simulink model "Control_v6_PID"  (R2020b)
settings: Solver=FixedStepAuto  StartTime=0.0  StopTime=t_sim  FixedStep=TimeStep  RelTol=1e-3
values from neighbouring files (symbols this model uses):
  date_IGRF = [date.year,date.month,date.day]    [main_SCA_v3.m]    (also in main_SCA_v3_alt.m; main_SCA_v4_LQR.m; main_SCA_v5.m)
  nmax = 2    [main_SCA.m]    (also in main_SCA_v3.m; main_SCA_v3_alt.m; main_SCA_v4_LQR.m; main_SCA_v5.m)
  Use_IGRF = 0    [main_SCA.m]    (also in main_SCA_v3.m; main_SCA_v3_alt.m; main_SCA_v4_LQR.m; main_SCA_v5.m = 1)
undefined symbols (not defined in the file or in its folder): att, date, deg, DipoleMod, DiscIntNeverNeededParam, IonSataero, km, orbit, rad, s, sat
libraries: vrlib x20, aerolibconvert2 x14, aerolibutil x14, dspmathops x13, sharedtransform x12, simulink x5, simulink_extras x2, dspstat3 x1, aerolibatmos2 x1, aerolibobsolete x1, sharedutil x1, aerolibcelestial x1
(part 1 of 3)
settings Model: EnablePacing=on  PacingRate=1000  Creator=colpari  LastModifiedBy=kang Shinok
settings OptimizationCC: DefaultParameterBehavior=Inlined  UseDivisionForNetSlopeComputation=on  GainParamInheritBuiltInType=on  UseFloatMulNetSlope=on  InlineInvariantSignals=on  EfficientFloat2IntCast=on  LifeSpan=1
settings HardwareCC: ProdLongLongMode=on
settings SFSimCC: MATLABDynamicMemAlloc=off
settings RTWCC: GenerateReport=on  LaunchReport=on
settings CodeAppCC: ForceParamTrailComments=on
settings GRTTargetCC: CombineSignalStateStructs=on  MatFileLogging=off  SupportVariableSizeSignals=on

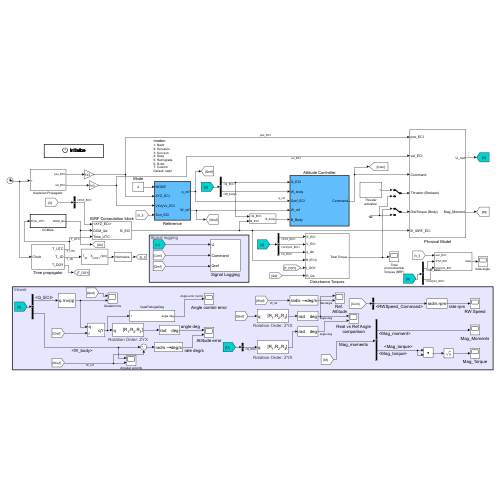
[thumbnail: Simulink's stored preview of the top-level diagram]
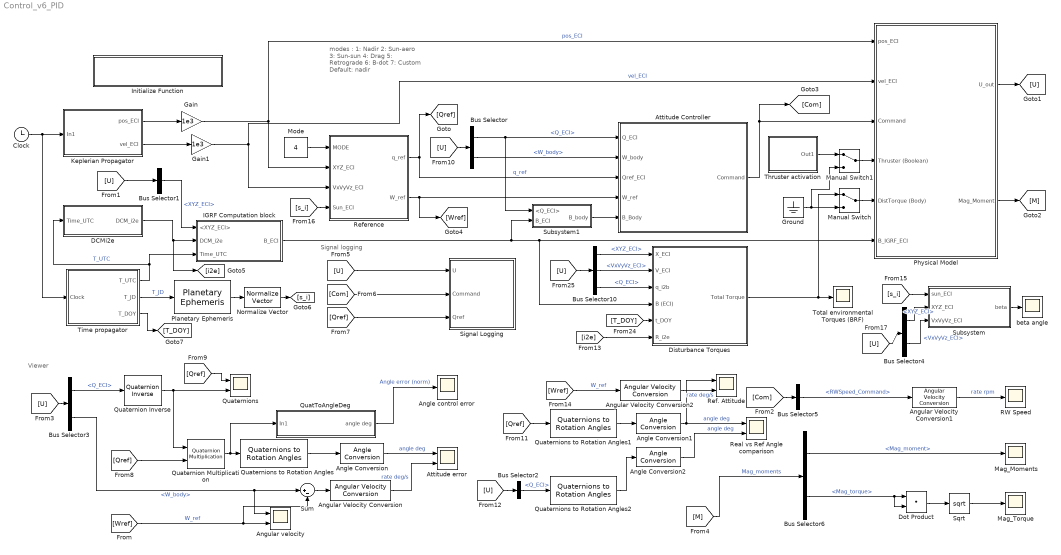
== system Control_v6_PID ==
  note: Viewer
  note: Signal logging
  note: modes :
      | 1: Nadir
      | 2: Sun-aero
      | 3: Sun-sun
      | 4: Drag
      | 5: Retrograde
      | 6: B-dot
      | 7: Custom
      | Default: nadir
  Angle Conversion : aerolibconvert2/Angle Conversion  IU=rad  OU=deg
  Angle Conversion1 : aerolibconvert2/Angle Conversion  IU=rad  OU=deg
  Angle Conversion2 : aerolibconvert2/Angle Conversion  IU=rad  OU=deg
  Angle control error : Scope
  Angular Velocity Conversion : aerolibconvert2/Angular Velocity Conversion  IU=rad/s  OU=deg/s
  Angular Velocity Conversion1 : aerolibconvert2/Angular Velocity Conversion  IU=rad/s  OU=rpm
  Angular Velocity Conversion2 : aerolibconvert2/Angular Velocity Conversion  IU=rad/s  OU=deg/s
  Angular velocity : Scope  NumInputPorts=2
  Attitude Controller : Subsystem  TreatAsAtomicUnit=on
  Attitude error : Scope  NumInputPorts=2
  Bus Selector : BusSelector  OutputSignals=Q_ECI,W_body
  Bus Selector1 : BusSelector  OutputSignals=XYZ_ECI
  Bus Selector10 : BusSelector  OutputSignals=XYZ_ECI,VxVyVz_ECI,Q_ECI
  Bus Selector2 : BusSelector  OutputSignals=Q_ECI
  Bus Selector3 : BusSelector  OutputSignals=Q_ECI,W_body
  Bus Selector4 : BusSelector  OutputSignals=XYZ_ECI,VxVyVz_ECI
  Bus Selector5 : BusSelector  OutputSignals=RWSpeed_Command
  Bus Selector6 : BusSelector  OutputSignals=Mag_moment,Mag_torque
  Clock : Clock
  DCMi2e : Subsystem  TreatAsAtomicUnit=on  SystemSampleTime=1
  Disturbance Torques : Subsystem
  Dot Product : DotProduct  InputSameDT=on  OutDataTypeStr=Inherit: Inherit via internal rule
  Gain : Gain  Gain=1e3
  Gain1 : Gain  Gain=1e3
  Ground : Ground
  IGRF Computation block : Subsystem
  Initialize Function : Subsystem  TreatAsAtomicUnit=on
  Keplerian Propagator : Subsystem
  Mag_Moments : Scope
  Mag_Torque : Scope
  Manual Switch : ManualSwitch
  Manual Switch1 : ManualSwitch
  Mode : Constant  Value=4  OutDataTypeStr=int8
  Normalize Vector : vrlib/Utilities/Normalize Vector  maxzero=0
  Physical Model : Subsystem
      settings: MinAlgLoopOccurrences=on
  Planetary Ephemeris : aerolibcelestial/Planetary Ephemeris  kmflag=km,km/s  epochflag=Julian date  de=DE405  nCenter=Earth  nTarget=Sun  errorflag=Error  velflag=off
      settings: SourceProductBaseCode=AE
  QuatToAngleDeg : Subsystem
  Quaternion Inverse : aerolibutil/Quaternion Inverse
  Quaternion Multiplication : aerolibutil/Quaternion Multiplication
  Quaternions : Scope  NumInputPorts=2
  Quaternions to Rotation Angles : sharedtransform/Quaternions to Rotation Angles  rotationOrder=ZYX  aMode=aMode
      settings: SourceProductBaseCode=AE,PW,DR,MT,UV,VE
  Quaternions to Rotation Angles1 : sharedtransform/Quaternions to Rotation Angles  rotationOrder=ZYX  aMode=aMode
      settings: SourceProductBaseCode=AE,PW,DR,MT,UV,VE
  Quaternions to Rotation Angles2 : sharedtransform/Quaternions to Rotation Angles  rotationOrder=ZYX  aMode=aMode
      settings: SourceProductBaseCode=AE,PW,DR,MT,UV,VE
  RW Speed : Scope
  Real vs Ref Angle comparison : Scope  NumInputPorts=2
  Ref. Attitude : Scope  NumInputPorts=2
  Reference : Subsystem  TreatAsAtomicUnit=on
  Signal Logging : Subsystem
  Sqrt : Sqrt  SaturateOnIntegerOverflow=on
  Subsystem : Subsystem
  Subsystem1 : Subsystem
  Sum : Sum  Inputs=|+-
  Thruster activation : Subsystem
  Time propagator : Subsystem
  Total environmental Torques (BRF) : Scope
  beta angle : Scope
  wires:
  Clock/1 -> Keplerian Propagator/1(In1), Time propagator/1(Clock)
  Keplerian Propagator/1(pos_ECI) -> Gain/1
  Keplerian Propagator/2(vel_ECI) -> Gain1/1
  Planetary Ephemeris/1 -> Normalize Vector/1
  Time propagator/2(T_JD) -> Planetary Ephemeris/1  "T_JD"
  Reference/1(q_ref) -> [Qref], Attitude Controller/3(Qref_ECI)  "q_ref"
  Physical Model/1(U_out) -> [U]
  Time propagator/1(T_UTC) -> DCMi2e/1(Time_UTC), IGRF Computation block/3("Time_UTC ")  "T_UTC"
  Gain/1 -> Reference/2(XYZ_ECI), Physical Model/1(pos_ECI)  "pos_ECI"
  Gain1/1 -> Reference/3(VxVyVz_ECI), Physical Model/2(vel_ECI)  "vel_ECI"
  Attitude Controller/1(Command) -> Physical Model/3(Command), [Com]
  IGRF Computation block/1(B_ECI) -> Subsystem1/2(B_ECI), Disturbance Torques/4(B (ECI)), Physical Model/6(B_IGRF_ECI)
  [U] -> Bus Selector/1
  Bus Selector/1 -> Subsystem1/1(<Q_ECI>), Attitude Controller/1(Q_ECI)  "<Q_ECI>"
  Bus Selector/2 -> Attitude Controller/2(W_body)  "<W_body>"
  [U] -> Bus Selector1/1
  Bus Selector1/1 -> IGRF Computation block/1(<XYZ_ECI>)  "<XYZ_ECI>"
  [Qref] -> Signal Logging/3(Qref)
  Quaternions to Rotation Angles/1 -> Angle Conversion/1
  Bus Selector6/2 -> Dot Product/2, Dot Product/1  "<Mag_torque>"
  Bus Selector6/1 -> Mag_Moments/1  "<Mag_moment>"
  Dot Product/1 -> Sqrt/1
  Bus Selector3/1 -> Quaternion Inverse/1  "<Q_ECI>"
  Sqrt/1 -> Mag_Torque/1
  Bus Selector5/1 -> Angular Velocity Conversion1/1  "<RWSpeed_Command>"
  [Com] -> Signal Logging/2(Command)
  [Com] -> Bus Selector5/1
  Bus Selector3/2 -> Sum/1, Angular velocity/1  "<W_body>"
  [Qref] -> Quaternion Multiplication/2
  [U] -> Bus Selector3/1
  Quaternion Inverse/1 -> Quaternion Multiplication/1, Quaternions/2
  [M] -> Bus Selector6/1  "Mag_moments"
  Angular Velocity Conversion/1 -> Attitude error/2  "rate deg/s"
  Quaternion Multiplication/1 -> QuatToAngleDeg/1(In1), Quaternions to Rotation Angles/1
  [U] -> Signal Logging/1(U)
  Angle Conversion/1 -> Attitude error/1  "angle deg"
  Angular Velocity Conversion1/1 -> RW Speed/1  "rate rpm"
  Physical Model/2(Mag_Moment) -> [M]
  Subsystem1/1(B_body) -> Attitude Controller/5(B_Body)
  QuatToAngleDeg/1(angle deg) -> Angle control error/1  "Angle error (norm)"
  [Qref] -> Quaternions/1
  Reference/2(W_ref) -> [Wref], Attitude Controller/4(W_ref)
  [Wref] -> Sum/2, Angular velocity/2  "W_ref"
  Sum/1 -> Angular Velocity Conversion/1
  [Qref] -> Quaternions to Rotation Angles1/1
  Angle Conversion1/1 -> Ref. Attitude/1, Real vs Ref Angle comparison/1  "angle deg"
  Quaternions to Rotation Angles1/1 -> Angle Conversion1/1
  Thruster activation/1(Out1) -> Manual Switch1/1
  [U] -> Bus Selector10/1
  [T_DOY] -> Disturbance Torques/5(t_DOY)
  Bus Selector10/3 -> Disturbance Torques/3(q_i2b)  "<Q_ECI>"
  Time propagator/3(T_DOY) -> [T_DOY]
  Disturbance Torques/1("Total Torque ") -> Total environmental Torques (BRF)/1, Manual Switch/1
  Manual Switch/1 -> Physical Model/5(DistTorque (Body))
  Ground/1 -> Manual Switch/2, Manual Switch1/2
  Bus Selector2/1 -> Quaternions to Rotation Angles2/1  "<Q_ECI>"
  Quaternions to Rotation Angles2/1 -> Angle Conversion2/1
  Angle Conversion2/1 -> Real vs Ref Angle comparison/2  "angle deg"
  [U] -> Bus Selector2/1
  [Wref] -> Angular Velocity Conversion2/1  "W_ref"
  Angular Velocity Conversion2/1 -> Ref. Attitude/2  "rate deg/s"
  DCMi2e/1(DCM_i2e) -> [i2e], IGRF Computation block/2("DCM_i2e ")
  [i2e] -> Disturbance Torques/6(R_i2e)
  Bus Selector10/1 -> Disturbance Torques/1(X_ECI)  "<XYZ_ECI>"
  Bus Selector10/2 -> Disturbance Torques/2(V_ECI)  "<VxVyVz_ECI>"
  Manual Switch1/1 -> Physical Model/4(Thruster (Boolean))
  Mode/1 -> Reference/1(MODE)
  [s_i] -> Subsystem/1(sun_ECI)
  Subsystem/1(beta) -> beta angle/1
  Normalize Vector/1 -> [s_i]
  [s_i] -> Reference/4(Sun_ECI)
  [U] -> Bus Selector4/1
  Bus Selector4/1 -> Subsystem/2(XYZ_ECI)  "<XYZ_ECI>"
  Bus Selector4/2 -> Subsystem/3(VxVyVz_ECI)  "<VxVyVz_ECI>"

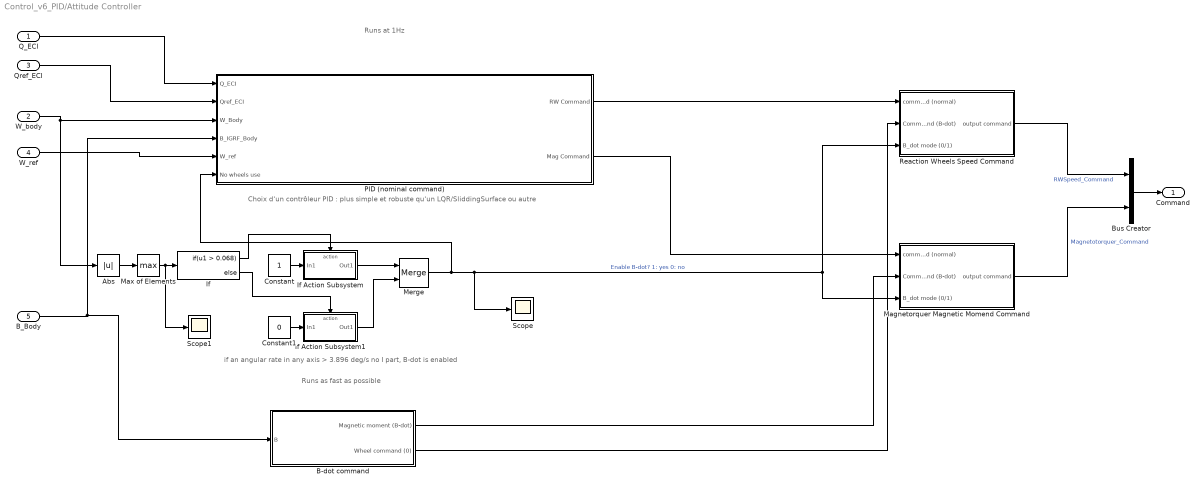
== system Control_v6_PID/Attitude Controller ==
  note: Choix d'un contrôleur PID : plus simple et robuste qu'un LQR/SliddingSurface ou autre
  note: Runs as fast as possible
  note: Runs at 1Hz
  note: if an angular rate in any axis > 3.896 deg/s no I part, B-dot is enabled
  Q_ECI : Inport
  W_body : Inport  Port=2
  Qref_ECI : Inport  Port=3
  W_ref : Inport  Port=4
  B_Body : Inport  Port=5
  Abs : Abs
  B-dot command : Subsystem  TreatAsAtomicUnit=on
  Bus Creator : BusCreator  Inputs=2
  Constant : Constant
  Constant1 : Constant  Value=0
  If : If  IfExpression=u1 > 0.068
  If Action Subsystem : Subsystem  TreatAsAtomicUnit=on
  If Action Subsystem1 : Subsystem  TreatAsAtomicUnit=on
  Magnetorquer Magnetic Momend Command : Subsystem
  Max of Elements : MinMax  Function=max
  Merge : Merge
  PID (nominal command) : Subsystem  TreatAsAtomicUnit=on  SystemSampleTime=1
  Reaction Wheels Speed Command : Subsystem
  Scope : Scope
  Scope1 : Scope
  Command : Outport  VectorParamsAs1DForOutWhenUnconnected=off
  wires:
  B_Body/1 -> B-dot command/1(B), PID (nominal command)/4(B_IGRF_Body)
  Magnetorquer Magnetic Momend Command/1(output command) -> Bus Creator/2  "Magnetotorquer_Command"
  Reaction Wheels Speed Command/1(output command) -> Bus Creator/1  "RWSpeed_Command"
  B-dot command/2(Wheel command (0)) -> Reaction Wheels Speed Command/2(Command (B-dot))
  B-dot command/1(Magnetic moment (B-dot)) -> Magnetorquer Magnetic Momend Command/2(Command (B-dot))
  Q_ECI/1 -> PID (nominal command)/1(Q_ECI)
  Qref_ECI/1 -> PID (nominal command)/2(Qref_ECI)
  PID (nominal command)/1(RW Command) -> Reaction Wheels Speed Command/1(" command (normal)")
  PID (nominal command)/2(Mag Command) -> Magnetorquer Magnetic Momend Command/1(" command (normal)")
  Bus Creator/1 -> Command/1
  Abs/1 -> Max of Elements/1
  If/1 -> If Action Subsystem/Action
  If Action Subsystem1/1(Out1) -> Merge/2
  Max of Elements/1 -> Scope1/1, If/1
  If/2 -> If Action Subsystem1/Action
  If Action Subsystem/1(Out1) -> Merge/1
  Constant/1 -> If Action Subsystem/1(In1)
  Merge/1 -> Scope/1, Magnetorquer Magnetic Momend Command/3(B_dot mode (0/1)), Reaction Wheels Speed Command/3(B_dot mode (0/1)), PID (nominal command)/6(No wheels use)  "Enable B-dot? 1: yes 0: no"
  Constant1/1 -> If Action Subsystem1/1(In1)
  W_body/1 -> Abs/1, PID (nominal command)/3(W_Body)
  W_ref/1 -> PID (nominal command)/5(W_ref)

== system Control_v6_PID/DCMi2e ==
  note: Slower subsytem because it's too slow
  Time_UTC : Inport
  ECI to ECEF : MATLABFcn  MATLABFcn=eci2ecef  OutputDimensions=[3;3]  Output1D=off
  DCM_i2e : Outport
  wires:
  ECI to ECEF/1 -> DCM_i2e/1
  Time_UTC/1 -> ECI to ECEF/1

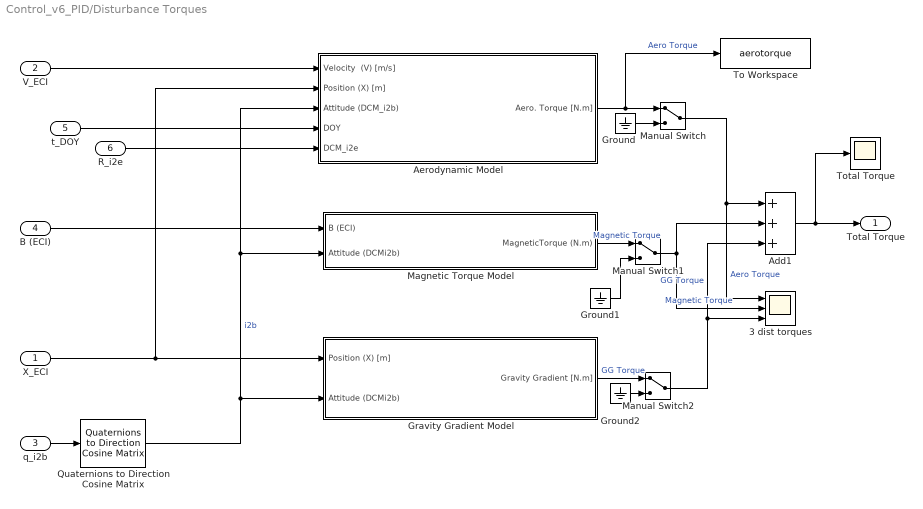
== system Control_v6_PID/Disturbance Torques ==
  X_ECI : Inport
  V_ECI : Inport  Port=2
  q_i2b : Inport  Port=3
  B (ECI) : Inport  Port=4
  t_DOY : Inport  Port=5
  R_i2e : Inport  Port=6
  3 dist torques : Scope  NumInputPorts=3
  Add1 : Sum  Inputs=+++
  Aerodynamic Model : Subsystem
  Gravity Gradient Model : Subsystem
  Ground : Ground
  Ground1 : Ground
  Ground2 : Ground
  Magnetic Torque Model : Subsystem
  Manual Switch : ManualSwitch
  Manual Switch1 : ManualSwitch
  Manual Switch2 : ManualSwitch
  Quaternions to Direction Cosine Matrix : sharedtransform/Quaternions to  Direction Cosine Matrix  aMode=aMode
      settings: SourceProductBaseCode=AE,PW,DR,MT,UV,VE
  To Workspace : ToWorkspace  VariableName=aerotorque  SaveFormat=Timeseries  SampleTime=-1
  Total Torque : Scope
  "Total Torque " : Outport
  wires:
  Add1/1 -> Total Torque/1, "Total Torque "/1
  V_ECI/1 -> Aerodynamic Model/1(Velocity  (V) [m/s])
  X_ECI/1 -> Aerodynamic Model/2(Position (X) [m]), Gravity Gradient Model/1("Position (X) [m] ")
  Manual Switch/1 -> 3 dist torques/1, Add1/1  "Aero Torque"
  Manual Switch2/1 -> Add1/3, 3 dist torques/3  "GG Torque"
  B (ECI)/1 -> Magnetic Torque Model/1(B (ECI))
  Manual Switch1/1 -> Add1/2, 3 dist torques/2  "Magnetic Torque"
  q_i2b/1 -> Quaternions to Direction Cosine Matrix/1
  Quaternions to Direction Cosine Matrix/1 -> Gravity Gradient Model/2(Attitude (DCMi2b)), Magnetic Torque Model/2(Attitude (DCMi2b)), Aerodynamic Model/3(Attitude (DCM_i2b))  "i2b"
  R_i2e/1 -> Aerodynamic Model/5(DCM_i2e)
  t_DOY/1 -> Aerodynamic Model/4(DOY)
  Ground/1 -> Manual Switch/2
  Aerodynamic Model/1(Aero. Torque [N.m]) -> To Workspace/1, Manual Switch/1  "Aero Torque"
  Magnetic Torque Model/1(MagneticTorque (N.m)) -> Manual Switch1/1  "Magnetic Torque"
  Ground1/1 -> Manual Switch1/2
  Ground2/1 -> Manual Switch2/2
  Gravity Gradient Model/1(Gravity Gradient [N.m]) -> Manual Switch2/1  "GG Torque"

== system Control_v6_PID/IGRF Computation block ==
  <XYZ_ECI> : Inport
  "DCM_i2e " : Inport  Port=2
  "Time_UTC " : Inport  Port=3
  Bus Creator : BusCreator  Inputs=5
  Bus Selector4 : BusSelector  OutputSignals=XYZ_ECI
  Constant : Constant  Value=[0.4;0.4;0.4]
  Cross Product : vrlib/Utilities/Cross Product
  Demux : Demux  Outputs=2
  ECI To LLA : MATLAB Function  TreatAsAtomicUnit=on
  MATLAB Function : MATLAB Function  TreatAsAtomicUnit=on
  Mux : Mux  Inputs=3
  Obtain B_ECI : Subsystem
  Product : Product  Multiplication=Matrix(*)
  Reshape : Reshape  OutputDimensionality=Row vector (2-D)
  Scope : Scope
  Terminator : Terminator
  To Workspace : ToWorkspace  VariableName=B_ECI  SaveFormat=Timeseries  SampleTime=-1
  B_ECI : Outport  VectorParamsAs1DForOutWhenUnconnected=off
  wires:
  ECI To LLA/3(long) -> Bus Creator/3
  ECI To LLA/2(lat) -> Bus Creator/2
  ECI To LLA/1(h) -> Bus Creator/1
  Demux/1 -> Bus Creator/4  "time_UTC"
  Demux/2 -> Terminator/1
  "DCM_i2e "/1 -> Product/2, Bus Creator/5  "DCM_i2e"
  <XYZ_ECI>/1 -> Bus Selector4/1
  Reshape/1 -> Product/1
  Product/1 -> ECI To LLA/1(X_ECEF)
  Bus Selector4/1 -> Reshape/1  "<XYZ_ECI>"
  Bus Creator/1 -> Obtain B_ECI/1(In1)
  Obtain B_ECI/1(u) -> Cross Product/2, MATLAB Function/1(u), Mux/1, To Workspace/1, B_ECI/1
  "Time_UTC "/1 -> Demux/1
  Mux/1 -> Scope/1
  MATLAB Function/1(y) -> Mux/2
  Constant/1 -> Cross Product/1
  Cross Product/1 -> Mux/3

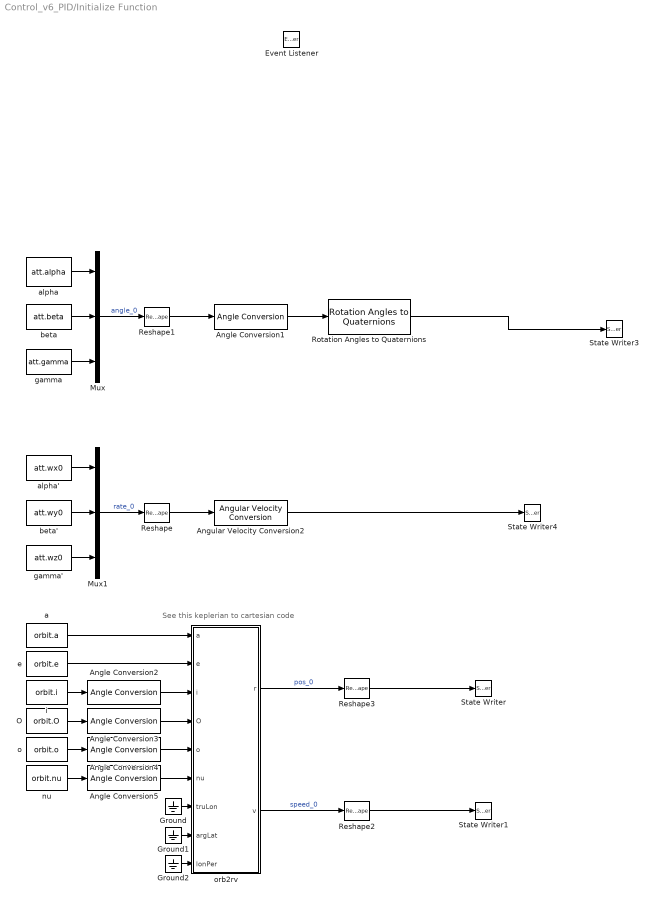
== system Control_v6_PID/Initialize Function ==
  note: See this keplerian to cartesian code
  Angle Conversion{1..5} (5 alike) : aerolibconvert2/Angle Conversion  IU=deg  OU=rad
  Angular Velocity Conversion2 : aerolibconvert2/Angular Velocity Conversion  IU=deg/s  OU=rad/s
  Event Listener : EventListener  DisableCoverage=on  EventName=reset
  Ground : Ground
  Ground1 : Ground
  Ground2 : Ground
  Mux : Mux  Inputs=3
  Mux1 : Mux  Inputs=3
  O : Constant  Value=orbit.O
  Reshape{,1..3} (4 alike) : Reshape  OutputDimensionality=Column vector (2-D)
  Rotation Angles to Quaternions : sharedtransform/Rotation Angles to Quaternions  rotationOrder=ZYX  aMode=aMode
      settings: SourceProductBaseCode=AE,PW,DR,MT,UV,VE
  State Writer : StateWriter  StateOwnerBlock=../../Keplerian Propagator/Integrator
  State Writer1 : StateWriter  StateOwnerBlock=../../Keplerian Propagator/Integrator1
  State Writer3 : StateWriter  StateOwnerBlock=../../Physical Model/6DOF in ECI frame/Compute Q_ECI/Integrator_quat
  State Writer4 : StateWriter  StateOwnerBlock=../../Physical Model/6DOF in ECI frame/Integrator_rate
  a : Constant  Value=orbit.a
  alpha : Constant  Value=att.alpha
  alpha' : Constant  Value=att.wx0
  beta : Constant  Value=att.beta
  beta' : Constant  Value=att.wy0
  e : Constant  Value=orbit.e
  gamma : Constant  Value=att.gamma
  gamma' : Constant  Value=att.wz0
  i : Constant  Value=orbit.i
  nu : Constant  Value=orbit.nu
  o : Constant  Value=orbit.o
  orb2rv : MATLAB Function  TreatAsAtomicUnit=on
  wires:
  Angular Velocity Conversion2/1 -> State Writer4/1
  Mux1/1 -> Reshape/1  "rate_0"
  Reshape/1 -> Angular Velocity Conversion2/1
  alpha'/1 -> Mux1/1
  gamma'/1 -> Mux1/3
  beta'/1 -> Mux1/2
  Reshape3/1 -> State Writer/1
  i/1 -> Angle Conversion2/1
  Ground/1 -> orb2rv/7(truLon)
  Angle Conversion2/1 -> orb2rv/3(i)
  nu/1 -> Angle Conversion5/1
  Ground2/1 -> orb2rv/9(lonPer)
  Angle Conversion3/1 -> orb2rv/4(O)
  Angle Conversion5/1 -> orb2rv/6(nu)
  Ground1/1 -> orb2rv/8(argLat)
  o/1 -> Angle Conversion4/1
  a/1 -> orb2rv/1(a)
  O/1 -> Angle Conversion3/1
  orb2rv/2(v) -> Reshape2/1  "speed_0"
  e/1 -> orb2rv/2(e)
  orb2rv/1(r) -> Reshape3/1  "pos_0"
  Angle Conversion4/1 -> orb2rv/5(o)
  Reshape2/1 -> State Writer1/1
  Reshape1/1 -> Angle Conversion1/1
  Angle Conversion1/1 -> Rotation Angles to Quaternions/1
  beta/1 -> Mux/2
  alpha/1 -> Mux/1
  gamma/1 -> Mux/3
  Mux/1 -> Reshape1/1  "angle_0"
  Rotation Angles to Quaternions/1 -> State Writer3/1

== system Control_v6_PID/Keplerian Propagator ==
  In1 : Inport
  Constant : Constant  Value=[0;0;0]
  Demux : Demux  Outputs=2
  Integrator : Integrator
  Integrator1 : Integrator
  Mux : Mux  Inputs=2
  Mux1 : Mux  Inputs=2
  Reshape1 : Reshape  OutputDimensionality=Customize  OutputDimensions=[6,1]
  Reshape3 : Reshape  OutputDimensionality=Column vector (2-D)
  keplerian propagator : MATLABFcn  MATLABFcn=kep_propagator
  pos_ECI : Outport
  vel_ECI : Outport  Port=2
  wires:
  Demux/2 -> vel_ECI/1  "vel_ECI"
  Demux/1 -> pos_ECI/1  "pos_ECI"
  keplerian propagator/1 -> Demux/1
  Mux1/1 -> keplerian propagator/1
  In1/1 -> Mux1/2
  Mux/1 -> Reshape1/1
  Reshape1/1 -> Mux1/1
  Integrator1/1 -> Mux/2
  Constant/1 -> Reshape3/1
  Reshape3/1 -> Integrator1/1, Integrator/1
  Integrator/1 -> Mux/1

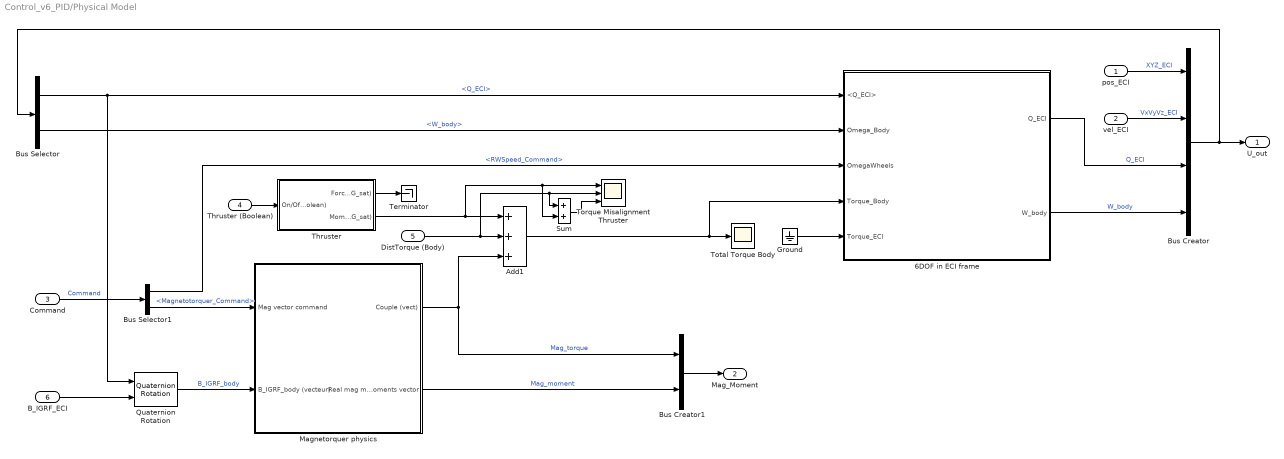
== system Control_v6_PID/Physical Model ==
  pos_ECI : Inport
  vel_ECI : Inport  Port=2
  Command : Inport  Port=3
  Thruster (Boolean) : Inport  Port=4
  DistTorque (Body) : Inport  Port=5
  B_IGRF_ECI : Inport  Port=6
  6DOF in ECI frame : Subsystem
  Add1 : Sum  Inputs=+++
  Bus Creator : BusCreator  Inputs=4
  Bus Creator1 : BusCreator  Inputs=2
  Bus Selector : BusSelector  OutputSignals=Q_ECI,W_body
  Bus Selector1 : BusSelector  OutputSignals=RWSpeed_Command,Magnetotorquer_Command
  Ground : Ground
  Magnetorquer physics : Subsystem
  Quaternion Rotation : aerolibutil/Quaternion Rotation
  Sum : Sum
  Terminator : Terminator
  Thruster : Subsystem
  Torque Misalignment Thruster : Scope  NumInputPorts=3
  Total Torque Body : Scope
  U_out : Outport  VectorParamsAs1DForOutWhenUnconnected=off
  Mag_Moment : Outport  Port=2  VectorParamsAs1DForOutWhenUnconnected=off
  wires:
  Thruster (Boolean)/1 -> Thruster/1(On/Off (Boolean))
  Bus Creator/1 -> U_out/1, Bus Selector/1
  Bus Selector/1 -> Quaternion Rotation/1, 6DOF in ECI frame/1(<Q_ECI>)  "<Q_ECI>"
  6DOF in ECI frame/1(Q_ECI) -> Bus Creator/3  "Q_ECI"
  Bus Selector1/2 -> Magnetorquer physics/1(Mag vector command)  "<Magnetotorquer_Command>"
  Thruster/2(Moment (G_sat)) -> Sum/2, Torque Misalignment Thruster/1, Add1/1
  Add1/1 -> Total Torque Body/1, 6DOF in ECI frame/4(Torque_Body)
  DistTorque (Body)/1 -> Sum/1, Torque Misalignment Thruster/2, Add1/2
  Bus Selector/2 -> 6DOF in ECI frame/2("Omega_Body ")  "<W_body>"
  B_IGRF_ECI/1 -> Quaternion Rotation/2
  Quaternion Rotation/1 -> Magnetorquer physics/2(B_IGRF_body (vecteur))  "B_IGRF_body"
  Magnetorquer physics/2(Real mag moments vector) -> Bus Creator1/2  "Mag_moment"
  Magnetorquer physics/1(Couple (vect)) -> Add1/3, Bus Creator1/1  "Mag_torque"
  6DOF in ECI frame/2(W_body) -> Bus Creator/4  "W_body"
  Command/1 -> Bus Selector1/1  "Command"
  Bus Selector1/1 -> 6DOF in ECI frame/3(OmegaWheels)  "<RWSpeed_Command>"
  Bus Creator1/1 -> Mag_Moment/1
  pos_ECI/1 -> Bus Creator/1  "XYZ_ECI"
  vel_ECI/1 -> Bus Creator/2  "VxVyVz_ECI"
  Thruster/1(Force (G_sat)) -> Terminator/1
  Ground/1 -> 6DOF in ECI frame/5(Torque_ECI)
  Sum/1 -> Torque Misalignment Thruster/3

== system Control_v6_PID/QuatToAngleDeg ==
  In1 : Inport
  Abs : Abs
  Angle Conversion1 : aerolibconvert2/Angle Conversion  IU=rad  OU=deg
  Demux1 : Demux
  Quaternion to axis and angle conversion : MATLABFcn  MATLABFcn=quat2axisangle
  Terminator1 : Terminator
  Terminator2 : Terminator
  Terminator3 : Terminator
  angle deg : Outport  VectorParamsAs1DForOutWhenUnconnected=off
  wires:
  Demux1/2 -> Terminator2/1
  Demux1/4 -> Angle Conversion1/1
  In1/1 -> Quaternion to axis and angle conversion/1
  Demux1/1 -> Terminator1/1
  Demux1/3 -> Terminator3/1
  Quaternion to axis and angle conversion/1 -> Demux1/1
  Abs/1 -> angle deg/1
  Angle Conversion1/1 -> Abs/1  "angle deg"

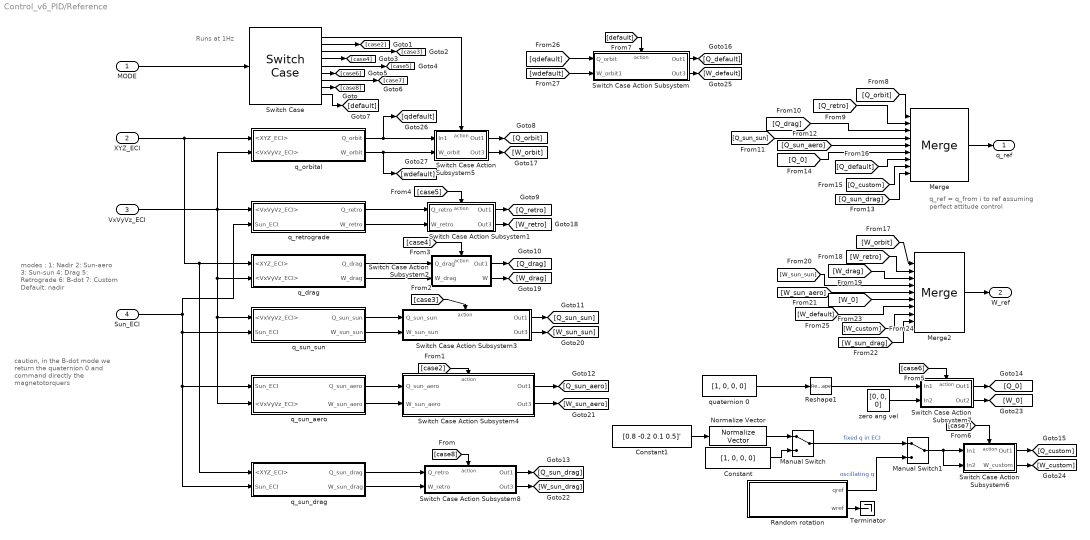
== system Control_v6_PID/Reference ==
  note: caution, in the B-dot mode we return the quaternion 0 and command directly the magnetotorquers
  note: modes :
      | 1: Nadir
      | 2: Sun-aero
      | 3: Sun-sun
      | 4: Drag
      | 5: Retrograde
      | 6: B-dot
      | 7: Custom
      | Default: nadir
  note: q_ref  = q_from i to ref
      | assuming perfect attitude control
  note: Runs at 1Hz
  MODE : Inport  OutMin=1  OutMax=100  OutDataTypeStr=int8
  XYZ_ECI : Inport  Port=2
  VxVyVz_ECI : Inport  Port=3
  Sun_ECI : Inport  Port=4
  Constant : Constant  Value=[1, 0, 0, 0]
  Constant1 : Constant  Value=[0.8 -0.2 0.1 0.5]'
  Manual Switch : ManualSwitch
  Manual Switch1 : ManualSwitch
  Merge : Merge  Inputs=9
  Merge2 : Merge  Inputs=9
  Normalize Vector : vrlib/Utilities/Normalize Vector  maxzero=0
  Random rotation : Subsystem
  Reshape1 : Reshape  OutputDimensionality=Column vector (2-D)
  Switch Case : SwitchCase  CaseConditions={1, 2, 3, 4, 5, 6, 7, 8}
  Switch Case Action Subsystem : Subsystem  TreatAsAtomicUnit=on
  Switch Case Action Subsystem1 : Subsystem  TreatAsAtomicUnit=on
  Switch Case Action Subsystem2 : Subsystem  TreatAsAtomicUnit=on
  Switch Case Action Subsystem3 : Subsystem  TreatAsAtomicUnit=on
  Switch Case Action Subsystem4 : Subsystem  TreatAsAtomicUnit=on
  Switch Case Action Subsystem5 : Subsystem  TreatAsAtomicUnit=on
  Switch Case Action Subsystem6 : Subsystem  TreatAsAtomicUnit=on
  Switch Case Action Subsystem7 : Subsystem  TreatAsAtomicUnit=on
  Switch Case Action Subsystem8 : Subsystem  TreatAsAtomicUnit=on
  Terminator : Terminator
  q_drag : Subsystem
  q_orbital : Subsystem
  q_retrograde : Subsystem
  q_sun_aero : Subsystem
  q_sun_drag : Subsystem
  q_sun_sun : Subsystem
  quaternion 0 : Constant  Value=[1, 0, 0, 0]
  zero ang vel : Constant  Value=[0, 0, 0]
  q_ref : Outport  VectorParamsAs1DForOutWhenUnconnected=off
  W_ref : Outport  Port=2
  wires:
  quaternion 0/1 -> Reshape1/1
  Reshape1/1 -> Switch Case Action Subsystem7/1(In1)
  Constant/1 -> Manual Switch/2
  Constant1/1 -> Normalize Vector/1
  Normalize Vector/1 -> Manual Switch/1
  zero ang vel/1 -> Switch Case Action Subsystem7/2(In2)
  Manual Switch/1 -> Manual Switch1/1  "fixed q in ECI"
  Random rotation/1(qref) -> Manual Switch1/2  "oscillating q"
  Manual Switch1/1 -> Switch Case Action Subsystem6/2(In2), Switch Case Action Subsystem6/1(In1)
  XYZ_ECI/1 -> q_sun_drag/1(<XYZ_ECI>), q_drag/1(<XYZ_ECI>), q_orbital/1(<XYZ_ECI>)
  [default] -> Switch Case Action Subsystem/Action
  Switch Case/7 -> [case7]
  Switch Case/4 -> [case4]
  Switch Case/5 -> [case5]
  [case3] -> Switch Case Action Subsystem3/Action
  [case5] -> Switch Case Action Subsystem1/Action
  Switch Case/3 -> [case3]
  Switch Case/2 -> [case2]
  q_drag/2(W_drag) -> Switch Case Action Subsystem2/2(W_drag)
  q_sun_drag/2(W_sun_drag) -> Switch Case Action Subsystem8/2(W_retro)
  q_sun_aero/2(W_sun_aero) -> Switch Case Action Subsystem4/2(W_sun_aero)
  Switch Case/1 -> Switch Case Action Subsystem5/Action
  [case8] -> Switch Case Action Subsystem8/Action
  Switch Case/8 -> [case8]
  q_drag/1(Q_drag) -> Switch Case Action Subsystem2/1(Q_drag)
  Switch Case/9 -> [default]
  Sun_ECI/1 -> q_retrograde/2(Sun_ECI), q_sun_drag/2(Sun_ECI), q_sun_aero/1(Sun_ECI), q_sun_sun/2(Sun_ECI)
  q_sun_sun/2(W_sun_sun) -> Switch Case Action Subsystem3/2(W_sun_sun)
  q_retrograde/2(W_retro) -> Switch Case Action Subsystem1/2(W_retro)
  q_sun_sun/1(Q_sun_sun) -> Switch Case Action Subsystem3/1(Q_sun_sun)
  q_sun_aero/1(Q_sun_aero) -> Switch Case Action Subsystem4/1(Q_sun_aero)
  q_sun_drag/1(Q_sun_drag) -> Switch Case Action Subsystem8/1(Q_retro)
  Merge2/1 -> W_ref/1
  [case2] -> Switch Case Action Subsystem4/Action
  [case4] -> Switch Case Action Subsystem2/Action
  q_orbital/1(Q_orbit) -> [qdefault], Switch Case Action Subsystem5/1(In1)
  q_retrograde/1(Q_retro) -> Switch Case Action Subsystem1/1(Q_retro)
  q_orbital/2(W_orbit) -> [wdefault], Switch Case Action Subsystem5/2(W_orbit)
  Switch Case/6 -> [case6]
  VxVyVz_ECI/1 -> q_orbital/2(<VxVyVz_ECI>), q_retrograde/1(<VxVyVz_ECI>), q_drag/2(<VxVyVz_ECI>), q_sun_aero/2(<VxVyVz_ECI>), q_sun_sun/1(<VxVyVz_ECI>)
  Merge/1 -> q_ref/1
  MODE/1 -> Switch Case/1
  Random rotation/2(wref) -> Terminator/1
  [case6] -> Switch Case Action Subsystem7/Action
  [case7] -> Switch Case Action Subsystem6/Action
  Switch Case Action Subsystem5/1(Out1) -> [Q_orbit]
  [Q_orbit] -> Merge/1
  Switch Case Action Subsystem1/1(Out1) -> [Q_retro]
  [Q_retro] -> Merge/2
  Switch Case Action Subsystem2/1(Out1) -> [Q_drag]
  [Q_drag] -> Merge/3
  Switch Case Action Subsystem3/1(Out1) -> [Q_sun_sun]
  [Q_sun_sun] -> Merge/4
  Switch Case Action Subsystem4/1(Out1) -> [Q_sun_aero]
  [Q_sun_aero] -> Merge/5
  Switch Case Action Subsystem8/1(Out1) -> [Q_sun_drag]
  [Q_sun_drag] -> Merge/9
  Switch Case Action Subsystem7/1(Out1) -> [Q_0]
  [Q_0] -> Merge/6
  Switch Case Action Subsystem6/1(Out1) -> [Q_custom]
  [Q_custom] -> Merge/8
  Switch Case Action Subsystem/1(Out1) -> [Q_default]
  [Q_default] -> Merge/7
  Switch Case Action Subsystem5/2(Out3) -> [W_orbit]
  [W_orbit] -> Merge2/1
  Switch Case Action Subsystem1/2(Out3) -> [W_retro]
  [W_retro] -> Merge2/2
  Switch Case Action Subsystem2/2(W) -> [W_drag]
  [W_drag] -> Merge2/3
  Switch Case Action Subsystem3/2(Out3) -> [W_sun_sun]
  [W_sun_sun] -> Merge2/4
  Switch Case Action Subsystem4/2(Out3) -> [W_sun_aero]
  [W_sun_aero] -> Merge2/5
  Switch Case Action Subsystem8/2(Out3) -> [W_sun_drag]
  [W_sun_drag] -> Merge2/9
  Switch Case Action Subsystem7/2(Out2) -> [W_0]
  [W_0] -> Merge2/6
  Switch Case Action Subsystem6/2(W_custom) -> [W_custom]
  [W_custom] -> Merge2/8
  Switch Case Action Subsystem/2(Out3) -> [W_default]
  [W_default] -> Merge2/7
  [qdefault] -> Switch Case Action Subsystem/1(Q_orbit)
  [wdefault] -> Switch Case Action Subsystem/2(W_orbit1)

== system Control_v6_PID/Signal Logging ==
  U : Inport
  Command : Inport  Port=2
  Qref : Inport  Port=3
  Bus Selector : BusSelector  OutputSignals=RWSpeed_Command,Magnetotorquer_Command
  Bus Selector4 : BusSelector  OutputSignals=XYZ_ECI,VxVyVz_ECI,Q_ECI,W_body
  Reshape : Reshape
  Reshape1 : Reshape
  Reshape2 : Reshape
  To Workspace : ToWorkspace  VariableName=sat_pos  SaveFormat=Timeseries  SampleTime=1
      settings: Save2DSignal=2-D array (concatenate along first dimension)
  To Workspace1 : ToWorkspace  VariableName=sat_speed  SaveFormat=Timeseries  SampleTime=1
      settings: Save2DSignal=2-D array (concatenate along first dimension)
  To Workspace2 : ToWorkspace  VariableName=sat_Q  SaveFormat=Timeseries  SampleTime=1
      settings: Save2DSignal=2-D array (concatenate along first dimension)
  To Workspace3 : ToWorkspace  VariableName=sat_omega  SaveFormat=Timeseries  SampleTime=1
      settings: Save2DSignal=2-D array (concatenate along first dimension)
  To Workspace4 : ToWorkspace  VariableName=RWSpeed_Command  SaveFormat=Timeseries  SampleTime=1
      settings: Save2DSignal=2-D array (concatenate along first dimension)
  To Workspace5 : ToWorkspace  VariableName=sat_Qc  SaveFormat=Timeseries  SampleTime=1
      settings: Save2DSignal=2-D array (concatenate along first dimension)
  To Workspace6 : ToWorkspace  VariableName=Mag_Command  SaveFormat=Timeseries  SampleTime=1
      settings: Save2DSignal=2-D array (concatenate along first dimension)
  wires:
  Bus Selector4/3 -> To Workspace2/1  "<Q_ECI>"
  Bus Selector4/4 -> To Workspace3/1  "<W_body>"
  U/1 -> Bus Selector4/1
  Bus Selector4/2 -> To Workspace1/1  "<VxVyVz_ECI>"
  Command/1 -> Bus Selector/1
  Bus Selector4/1 -> To Workspace/1  "<XYZ_ECI>"
  Qref/1 -> Reshape1/1
  Reshape/1 -> To Workspace4/1
  Reshape1/1 -> To Workspace5/1
  Bus Selector/1 -> Reshape/1  "<RWSpeed_Command>"
  Bus Selector/2 -> Reshape2/1  "<Magnetotorquer_Command>"
  Reshape2/1 -> To Workspace6/1

== system Control_v6_PID/Subsystem ==
  sun_ECI : Inport
  XYZ_ECI : Inport  Port=2
  VxVyVz_ECI : Inport  Port=3
  Acos : Trigonometry  Operator=acos
  Constant1 : Constant  Value=90
  Cross Product : vrlib/Utilities/Cross Product
  Dot Product1 : DotProduct  InputSameDT=on  OutDataTypeStr=Inherit: Inherit via internal rule
  Gain2 : Gain  Gain=180/pi
  Normalize Vector2 : vrlib/Utilities/Normalize Vector  maxzero=0
  Sum1 : Sum  Inputs=|-+
  beta : Outport
  wires:
  Constant1/1 -> Sum1/2
  Acos/1 -> Gain2/1
  Dot Product1/1 -> Acos/1
  Cross Product/1 -> Normalize Vector2/1
  Gain2/1 -> Sum1/1
  VxVyVz_ECI/1 -> Cross Product/2
  XYZ_ECI/1 -> Cross Product/1  "pos_ECI"
  Normalize Vector2/1 -> Dot Product1/2  "x"
  sun_ECI/1 -> Dot Product1/1
  Sum1/1 -> beta/1

== system Control_v6_PID/Subsystem1 ==
  <Q_ECI> : Inport
  B_ECI : Inport  Port=2
  Quaternion Rotation : aerolibutil/Quaternion Rotation
  B_body : Outport
  wires:
  <Q_ECI>/1 -> Quaternion Rotation/1
  B_ECI/1 -> Quaternion Rotation/2
  Quaternion Rotation/1 -> B_body/1  "B_IGRF_body"

== system Control_v6_PID/Thruster activation ==
  Clock1 : Clock
  Constant3 : Constant  Value=sat.thruster.duration
  Constant4 : Constant  Value=sat.thruster.firstimpulse
  Constant5 : Constant  Value=sat.thruster.wait
  Constant6 : Constant  Value=sat.thruster.Nfirings
  MATLAB Function : MATLAB Function  TreatAsAtomicUnit=on
  Mux1 : Mux  Inputs=5
  Scope : Scope
  Out1 : Outport  VectorParamsAs1DForOutWhenUnconnected=off
  wires:
  MATLAB Function/1(y) -> Scope/1, Out1/1
  Clock1/1 -> Mux1/1
  Constant4/1 -> Mux1/3
  Constant6/1 -> Mux1/5
  Mux1/1 -> MATLAB Function/1(u)
  Constant3/1 -> Mux1/2
  Constant5/1 -> Mux1/4

== system Control_v6_PID/Time propagator ==
  note: Time initialization
  Clock : Inport
  Add : Sum  Inputs=|++
  Constant : Constant  Value=86400
  Day : Constant  Value=date.day
  Divide : Product  Inputs=*/
  HH : Constant  Value=date.hours
  JD to UTC : MATLAB Function  TreatAsAtomicUnit=on
  MATLAB Function : MATLAB Function  TreatAsAtomicUnit=on
  MM : Constant  Value=date.minutes
  Month : Constant  Value=date.month
  Mux : Mux  Inputs=6
  Mux1 : Mux  Inputs=3
  Reshape : Reshape
  SS : Constant  Value=date.seconds
  Signal logging : ToWorkspace  VariableName=T_UTC  SaveFormat=Timeseries  SampleTime=1
      settings: Save2DSignal=2-D array (concatenate along first dimension)
  Signal logging1 : ToWorkspace  VariableName=T_JD  SaveFormat=Timeseries  SampleTime=1
      settings: Save2DSignal=2-D array (concatenate along first dimension)
  UTC to JD : MATLAB Function  TreatAsAtomicUnit=on
  Year : Constant  Value=date.year
  T_UTC : Outport  VectorParamsAs1DForOutWhenUnconnected=off
  T_JD : Outport  Port=2  VectorParamsAs1DForOutWhenUnconnected=off
  T_DOY : Outport  Port=3
  wires:
  UTC to JD/1(JD) -> Add/1  "JD_0"
  Constant/1 -> Divide/2
  JD to UTC/1(Time_UTC) -> T_UTC/1, Reshape/1
  Divide/1 -> Add/2
  Mux/1 -> UTC to JD/1(Time_UTC)
  Day/1 -> Mux/3
  Month/1 -> Mux/2
  Year/1 -> Mux/1
  HH/1 -> Mux/4
  MM/1 -> Mux/5
  SS/1 -> Mux/6
  Reshape/1 -> Signal logging/1
  Add/1 -> Signal logging1/1, T_JD/1, JD to UTC/1(JD)
  MATLAB Function/1(Y) -> Mux1/1
  MATLAB Function/2(DOY) -> Mux1/2
  MATLAB Function/3(S) -> Mux1/3
  Mux1/1 -> T_DOY/1
  Clock/1 -> MATLAB Function/1(t), Divide/1

== system Control_v6_PID/Attitude Controller/B-dot command ==
  note: ref : OneDrive\IonSat X18\SCAO\Contrôle attitude\Detumbling\Detumbling and Aerostable Control for Cubesats.pdf
      |
      | formulae:
      | $\mathbf{\dot B} \simeq \mathbf{B}\times \mathbf{\dot \theta}$
      | $\mathbf{m} = -c\mathbf{\dot B}$
      |
      | this block does NOT decide if the B-dot mode is relevant or not
      | (it applies it without question on the rotation rate :
      | $\Omega=v/r= \sqrt{\frac{Gm_{earth}}{(h+r_{earth})^{3/2}}} \sim 0.066 °/s$ So the command MUST stop the B-dot mode when the estimated rotation speed is smaller than 0.1 degree per second )
  note: entrée:
      | champ magnétique
      | sortie: moment magnetique de commande et vitesse des roues à réaction (nulle)
  B : Inport
  Discrete Derivative : simulink/Discrete/Discrete Derivative  gainval=1.0  ICPrevScaledInput=0.0  OutMin=[]  OutMax=[]  OutDataType=fixdt(1, 16)  OutScaling=2^-10  DoSatur=off
  Divide1 : Product  Inputs=**
  Reshape2 : Reshape  OutputDimensionality=Column vector (2-D)
  constant c : Constant  Value=-sat.bdot_c
  wheels unused : Constant  Value=[0, 0, 0, 0]
  Magnetic moment (B-dot) : Outport  VectorParamsAs1DForOutWhenUnconnected=off
  Wheel command (0) : Outport  Port=2  VectorParamsAs1DForOutWhenUnconnected=off
  wires:
  constant c/1 -> Divide1/2
  B/1 -> Discrete Derivative/1
  Discrete Derivative/1 -> Divide1/1  "B_point=B^theta_point"
  Divide1/1 -> Magnetic moment (B-dot)/1
  wheels unused/1 -> Reshape2/1
  Reshape2/1 -> Wheel command (0)/1

== system Control_v6_PID/Attitude Controller/If Action Subsystem ==
  In1 : Inport
  Action Port : ActionPort  ActionPortLabel=if(u1 > 0.068)
  Out1 : Outport  VectorParamsAs1DForOutWhenUnconnected=off
  wires:
  In1/1 -> Out1/1

== system Control_v6_PID/Attitude Controller/If Action Subsystem1 ==
  In1 : Inport
  Action Port : ActionPort  ActionPortLabel=else
  Out1 : Outport  VectorParamsAs1DForOutWhenUnconnected=off
  wires:
  In1/1 -> Out1/1

== system Control_v6_PID/Attitude Controller/Magnetorquer Magnetic Momend Command ==
  " command (normal)" : Inport
  Command (B-dot) : Inport  Port=2
  B_dot mode (0/1) : Inport  Port=3
  If1 : If
  Merge : Merge
  Switch Case Action Subsystem3 : Subsystem  TreatAsAtomicUnit=on
  Switch Case Action Subsystem4 : Subsystem  TreatAsAtomicUnit=on
  output command : Outport  VectorParamsAs1DForOutWhenUnconnected=off
  wires:
  If1/2 -> Switch Case Action Subsystem4/Action
  If1/1 -> Switch Case Action Subsystem3/Action
  B_dot mode (0/1)/1 -> If1/1
  Command (B-dot)/1 -> Switch Case Action Subsystem3/1(In1)
  Switch Case Action Subsystem3/1(Out1) -> Merge/1
  Switch Case Action Subsystem4/1(Out1) -> Merge/2
  " command (normal)"/1 -> Switch Case Action Subsystem4/1(In1)
  Merge/1 -> output command/1

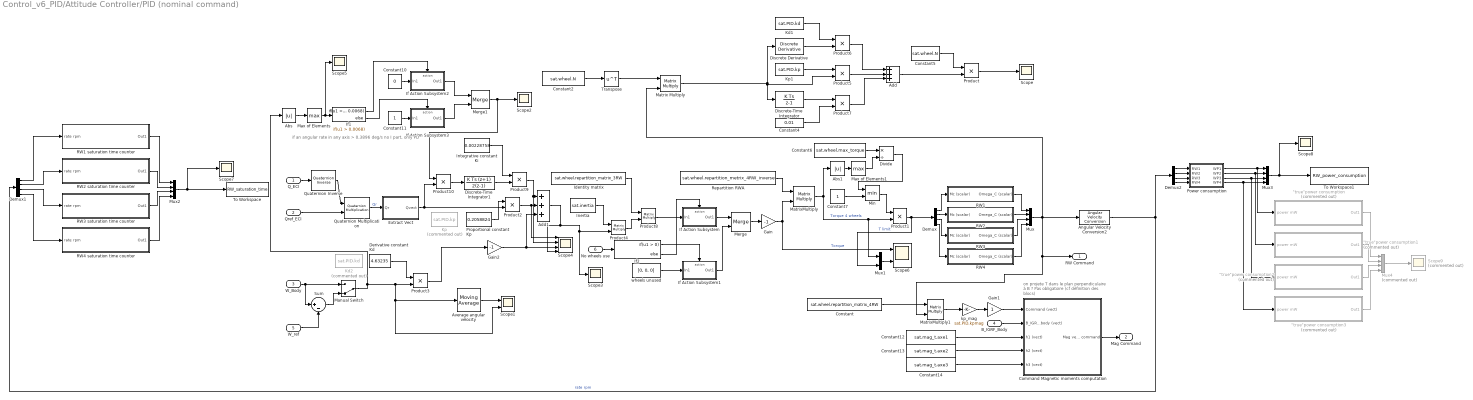
== system Control_v6_PID/Attitude Controller/PID (nominal command) ==
  note: if an angular rate in any axis > 0.3896 deg/s no I part, only PD
  note: on projete T dans
      | le plan perpendiculaire à B ?
      | Pas obligatoire (cf définition des blocs)
  Q_ECI : Inport
  Qref_ECI : Inport  Port=2
  W_Body : Inport  Port=3
  B_IGRF_Body : Inport  Port=4
  W_ref : Inport  Port=5
  No wheels use : Inport  Port=6
  "\"true\"power consumption" : Subsystem  Commented=on
  "\"true\"power consumption1" : Subsystem  Commented=on
  "\"true\"power consumption2" : Subsystem  Commented=on
  "\"true\"power consumption3" : Subsystem  Commented=on
  Abs : Abs
  Abs1 : Abs
  Add : Sum  Inputs=+++
  Add1 : Sum  Inputs=+++
  Angular Velocity Conversion2 : aerolibconvert2/Angular Velocity Conversion  IU=rad/s  OU=rpm
  Average angular velocity : dspstat3/Moving Average  Method=Sliding window  ForgettingFactorPort=off  SpecifyWindowLength=on  WindowLength=4  ForgettingFactor=0.9  SimulateUsing=Code generation
  Command Magnetic moments computation : Subsystem
  Constant : Constant  Value=sat.wheel.repartition_matrix_4RW
  Constant10 : Constant  Value=0
  Constant11 : Constant
  Constant12 : Constant  Value=sat.mag_t.axe1
  Constant13 : Constant  Value=sat.mag_t.axe2
  Constant14 : Constant  Value=sat.mag_t.axe3
  Constant2 : Constant  Value=sat.wheel.N
  Constant4 : Constant  Value=0.01
  Constant5 : Constant  Value=sat.wheel.N
  Constant6 : Constant  Value=sat.wheel.max_torque
  Constant7 : Constant
  Demux : Demux
  Demux1 : Demux
  Demux2 : Demux
  Derivative constant Kd : Constant  Value=4.63235
  Discrete Derivative : simulink/Discrete/Discrete Derivative  gainval=1.0  ICPrevScaledInput=0.0  OutMin=[]  OutMax=[]  OutDataType=fixdt(1, 16)  OutScaling=2^-10  DoSatur=off
  Discrete-Time Integrator : DiscreteIntegrator  SampleTime=-1  ICPrevOutput=DiscIntNeverNeededParam  ICPrevScaledInput=DiscIntNeverNeededParam
  Discrete-Time Integrator1 : DiscreteIntegrator  IntegratorMethod=Integration: Trapezoidal  SampleTime=-1  ICPrevOutput=DiscIntNeverNeededParam  ICPrevScaledInput=DiscIntNeverNeededParam
  Divide : Product  Inputs=*/
  Extract Vect : Subsystem
  Gain : Gain  Gain=-1
  Gain1 : Gain
  Gain2 : Gain  Gain=-1
  Identity matrix : Constant  Value=sat.wheel.repartition_matrix_3RW
  If Action Subsystem : Subsystem  TreatAsAtomicUnit=on
  If Action Subsystem1 : Subsystem  TreatAsAtomicUnit=on
  If Action Subsystem2 : Subsystem  TreatAsAtomicUnit=on
  If Action Subsystem3 : Subsystem  TreatAsAtomicUnit=on
  If1 : If  IfExpression=u1 > 0.0068
  If2 : If
  Inertia : Constant  Value=sat.inertia
  Integrative constant Ki : Constant  Value=0.00228758
  Kd1 : Constant  Value=sat.PID.kd
  Kd2 : Constant  Commented=on  Value=sat.PID.kd
  Kp : Constant  Commented=on  Value=sat.PID.kp
  Kp1 : Constant  Value=sat.PID.kp
  Manual Switch : ManualSwitch  CurrentSetting=0
  Matrix Multiply : Product  Multiplication=Matrix(*)
  MatrixMultiply : Product  Multiplication=Matrix(*)
  MatrixMultiply1 : Product  Multiplication=Matrix(*)
  Max of Elements : MinMax  Function=max
  Max of Elements1 : MinMax  Function=max
  Merge : Merge
  Merge1 : Merge
  Min : MinMax  Inputs=2
  Mux : Mux
  Mux1 : Mux  Inputs=2
  Mux2 : Mux
  Mux3 : Mux
  Mux4 : Mux  Commented=on
  Power consumption : MATLAB Function  TreatAsAtomicUnit=on
  Product{,1..3,5..7,9..10} (9 alike) : Product
  Product4 : Product  Multiplication=Matrix(*)
  Product8 : Product  Multiplication=Matrix(*)
  Proportional constant Kp : Constant  Value=0.2058824
  Quaternion Inverse : aerolibutil/Quaternion Inverse
  Quaternion Multiplication : aerolibutil/Quaternion Multiplication
  RW1 : Subsystem
  RW1 saturation time counter : Subsystem
  RW2 : Subsystem
  RW2 saturation time counter : Subsystem
  RW3 : Subsystem
  RW3 saturation time counter : Subsystem
  "RW4 " : Subsystem
  RW4 saturation time counter : Subsystem
  Repartition RWA : Constant  Value=sat.wheel.repartition_metrix_4RW_inverse
  Scope{,2..3,5,7..8} (6 alike) : Scope
  Scope1 : Scope  NumInputPorts=2
  Scope4 : Scope  NumInputPorts=4
  Scope6 : Scope  NumInputPorts=2
  Scope9 : Scope  Commented=on
  Sum : Sum  Inputs=|+-
  To Workspace : ToWorkspace  VariableName=RW_saturation_time  SaveFormat=Timeseries  SampleTime=-1
  To Workspace1 : ToWorkspace  VariableName=RW_power_consumption  SaveFormat=Timeseries  SampleTime=-1
  Transpose : Math  Operator=transpose  SaturateOnIntegerOverflow=on
  kp_mag : Gain  Gain=sat.PID.kpmag
  wheels unused : Constant  Value=[0, 0, 0]
  RW Command : Outport  VectorParamsAs1DForOutWhenUnconnected=off
  Mag Command : Outport  Port=2  VectorParamsAs1DForOutWhenUnconnected=off
  wires:
  Constant2/1 -> Transpose/1
  Kp1/1 -> Product5/1
  Discrete Derivative/1 -> Product6/2
  Kd1/1 -> Product6/1
  Discrete-Time Integrator/1 -> Product7/1
  Constant4/1 -> Product7/2
  Product6/1 -> Add/1
  Product5/1 -> Add/2
  Product7/1 -> Add/3
  Constant5/1 -> Product/1
  Add/1 -> Product/2
  Matrix Multiply/1 -> Discrete-Time Integrator/1, Product5/2, Discrete Derivative/1
  Transpose/1 -> Matrix Multiply/1
  Product/1 -> Scope/1
  No wheels use/1 -> If2/1
  MatrixMultiply/1 -> Abs1/1, Product1/2, Mux1/1  "Torque 4 wheels"
  Command Magnetic moments computation/1(Mag vector command) -> Mag Command/1
  Merge/1 -> Gain/1
  Product8/1 -> If Action Subsystem/1(In1)
  Constant14/1 -> Command Magnetic moments computation/5(h3 (vect))
  Constant12/1 -> Command Magnetic moments computation/3(h1 (vect))
  Constant/1 -> MatrixMultiply1/1
  Manual Switch/1 -> Abs/1, Scope1/2, Average angular velocity/1, Product3/2
  Constant11/1 -> If Action Subsystem3/1(In1)
  If2/2 -> If Action Subsystem/Action
  Max of Elements1/1 -> Divide/2
  Abs1/1 -> Max of Elements1/1
  Average angular velocity/1 -> Scope1/1
  Product10/1 -> Discrete-Time Integrator1/1
  Constant10/1 -> If Action Subsystem2/1(In1)
  Derivative constant Kd/1 -> Product3/1
  Demux/4 -> "RW4 "/1(Mc (scalar))
  Constant6/1 -> Divide/1
  Constant13/1 -> Command Magnetic moments computation/4(h2 (vect))
  Abs/1 -> Max of Elements/1
  Demux/3 -> RW3/1(Mc (scalar))
  Inertia/1 -> Product4/1
  RW3/1(Omega_C (scalar)) -> Mux/3
  Product9/1 -> Scope4/2, Add1/1
  RW2/1(Omega_C (scalar)) -> Mux/2
  Demux/2 -> RW2/1(Mc (scalar))
  Demux/1 -> RW1/1(Mc (scalar))
  If Action Subsystem/1(Out1) -> Merge/1
  If1/2 -> If Action Subsystem3/Action
  Constant7/1 -> Min/2
  If Action Subsystem3/1(Out1) -> Merge1/2
  If Action Subsystem2/1(Out1) -> Merge1/1
  Add1/1 -> Scope4/4, Scope3/1, Product4/2
  Identity matrix/1 -> Product8/1
  Gain1/1 -> Command Magnetic moments computation/1(Command (vect))
  Repartition RWA/1 -> MatrixMultiply/1
  Divide/1 -> Min/1
  Qref_ECI/1 -> Quaternion Multiplication/2
  wheels unused/1 -> If Action Subsystem1/1(In1)
  Max of Elements/1 -> Scope5/1, If1/1
  Merge1/1 -> Scope2/1, Product10/1
  Product4/1 -> Product8/2
  B_IGRF_Body/1 -> Command Magnetic moments computation/2(B_IGRF_body (vect))
  Q_ECI/1 -> Quaternion Inverse/1
  Product2/1 -> Scope4/1, Add1/2
  "RW4 "/1(Omega_C (scalar)) -> Mux/4
  Discrete-Time Integrator1/1 -> Product9/2
  Proportional constant Kp/1 -> Product2/1
  If1/1 -> If Action Subsystem2/Action
  If2/1 -> If Action Subsystem1/Action
  Quaternion Multiplication/1 -> Extract Vect/1(Qr)  "Qr"
  Extract Vect/1(Qvect) -> Product10/2, Product2/2
  Min/1 -> Product1/1
  Integrative constant Ki/1 -> Product9/1
  If Action Subsystem1/1(Out1) -> Merge/2
  Product1/1 -> Mux1/2, Demux/1  "T limit"
  Product3/1 -> Gain2/1
  kp_mag/1 -> Gain1/1
  Quaternion Inverse/1 -> Quaternion Multiplication/1
  MatrixMultiply1/1 -> kp_mag/1
  Gain/1 -> Scope6/1, MatrixMultiply/2  "Torque"
  W_Body/1 -> Sum/1, Manual Switch/1
  W_ref/1 -> Sum/2
  Sum/1 -> Manual Switch/2
  Gain2/1 -> Add1/3, Scope4/3
  Mux1/1 -> Scope6/2
  RW1/1(Omega_C (scalar)) -> Mux/1
  Demux1/1 -> RW1 saturation time counter/1(rate rpm)
  Demux1/4 -> RW4 saturation time counter/1(rate rpm)
  Mux/1 -> Matrix Multiply/2, Angular Velocity Conversion2/1, MatrixMultiply1/2, RW Command/1
  Demux1/3 -> RW3 saturation time counter/1(rate rpm)
  Demux1/2 -> RW2 saturation time counter/1(rate rpm)
  Angular Velocity Conversion2/1 -> Demux2/1, Demux1/1  "rate rpm"
  RW4 saturation time counter/1(Out1) -> Mux2/4
  RW2 saturation time counter/1(Out1) -> Mux2/2
  RW3 saturation time counter/1(Out1) -> Mux2/3
  RW1 saturation time counter/1(Out1) -> Mux2/1
  Mux2/1 -> Scope7/1, To Workspace/1
  Mux3/1 -> To Workspace1/1, Scope8/1
  Demux2/1 -> Power consumption/1(RW1)
  Demux2/2 -> Power consumption/2(RW2)
  Demux2/3 -> Power consumption/3(RW3)
  Demux2/4 -> Power consumption/4(RW4)
  Power consumption/2(WP2) -> "\"true\"power consumption1"/1(power mW), Mux3/2
  Power consumption/3(WP3) -> "\"true\"power consumption2"/1(power mW), Mux3/3
  Power consumption/4(WP4) -> "\"true\"power consumption3"/1(power mW), Mux3/4
  Power consumption/1(WP1) -> "\"true\"power consumption"/1(power mW), Mux3/1
  "\"true\"power consumption"/1(Out1) -> Mux4/1
  "\"true\"power consumption1"/1(Out1) -> Mux4/2
  "\"true\"power consumption2"/1(Out1) -> Mux4/3
  Mux4/1 -> Scope9/1
  "\"true\"power consumption3"/1(Out1) -> Mux4/4

== system Control_v6_PID/Attitude Controller/Reaction Wheels Speed Command ==
  " command (normal)" : Inport
  Command (B-dot) : Inport  Port=2
  B_dot mode (0/1) : Inport  Port=3
  If1 : If
  Merge : Merge
  Switch Case Action Subsystem3 : Subsystem  TreatAsAtomicUnit=on
  Switch Case Action Subsystem4 : Subsystem  TreatAsAtomicUnit=on
  output command : Outport  VectorParamsAs1DForOutWhenUnconnected=off
  wires:
  If1/2 -> Switch Case Action Subsystem4/Action
  If1/1 -> Switch Case Action Subsystem3/Action
  B_dot mode (0/1)/1 -> If1/1
  Command (B-dot)/1 -> Switch Case Action Subsystem3/1(In1)
  Merge/1 -> output command/1
  Switch Case Action Subsystem3/1(Out1) -> Merge/1
  Switch Case Action Subsystem4/1(Out1) -> Merge/2
  " command (normal)"/1 -> Switch Case Action Subsystem4/1(In1)

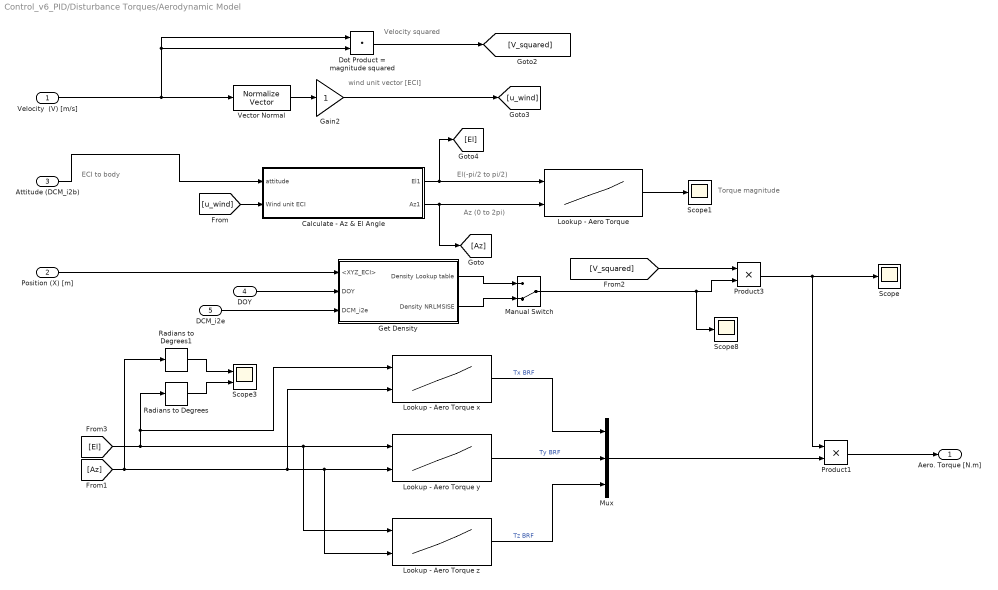
== system Control_v6_PID/Disturbance Torques/Aerodynamic Model ==
  note: Az (0 to 2pi)
  note: wind unit vector [ECI]
  note: Torque magnitude
  note: ECI to body
  note: Velocity squared
  note: El(-pi/2 to pi/2)
  Velocity  (V) [m/s] : Inport
  Position (X) [m] : Inport  Port=2
  Attitude (DCM_i2b) : Inport  Port=3
  DOY : Inport  Port=4
  DCM_i2e : Inport  Port=5
  Calculate - Az & El Angle : Subsystem
  Dot Product = magnitude squared : DotProduct  InputSameDT=on  OutDataTypeStr=Inherit: Inherit via internal rule
  Gain2 : Gain
  Get Density : Subsystem
  Lookup - Aero Torque : Lookup2D  RowIndex=IonSataero.Az  ColumnIndex=IonSataero.El  Table=IonSataero.T
  Lookup - Aero Torque x : Lookup2D  RowIndex=IonSataero.Az  ColumnIndex=IonSataero.El  Table=IonSataero.Tx
  Lookup - Aero Torque y : Lookup2D  RowIndex=IonSataero.Az  ColumnIndex=IonSataero.El  Table=IonSataero.Ty
  Lookup - Aero Torque z : Lookup2D  RowIndex=IonSataero.Az  ColumnIndex=IonSataero.El  Table=IonSataero.Tz
  Manual Switch : ManualSwitch  CurrentSetting=0
  Mux : Mux  Inputs=3
  Product1 : Product  RndMeth=Zero
  Product3 : Product  RndMeth=Zero
  Radians to Degrees : simulink_extras/Transformations/Radians to Degrees
  Radians to Degrees1 : simulink_extras/Transformations/Radians to Degrees
  Scope : Scope
  Scope1 : Scope
  Scope3 : Scope  NumInputPorts=2
  Scope8 : Scope
  Vector Normal : vrlib/Utilities/Normalize Vector  maxzero=0
  Aero. Torque [N.m] : Outport
  wires:
  Dot Product = magnitude squared/1 -> [V_squared]
  Vector Normal/1 -> Gain2/1
  Gain2/1 -> [u_wind]
  Lookup - Aero Torque/1 -> Scope1/1
  Attitude (DCM_i2b)/1 -> Calculate - Az & El Angle/1(attitude)
  [V_squared] -> Product3/1
  Velocity  (V) [m/s]/1 -> Dot Product = magnitude squared/2, Dot Product = magnitude squared/1, Vector Normal/1
  Radians to Degrees1/1 -> Scope3/1
  Radians to Degrees/1 -> Scope3/2
  [u_wind] -> Calculate - Az & El Angle/2(Wind unit ECI)
  Calculate - Az & El Angle/2(Az1) -> [Az], Lookup - Aero Torque/2
  Calculate - Az & El Angle/1(El1) -> [El], Lookup - Aero Torque/1
  [El] -> Lookup - Aero Torque z/1, Lookup - Aero Torque y/1, Lookup - Aero Torque x/1, Radians to Degrees/1
  [Az] -> Radians to Degrees1/1, Lookup - Aero Torque z/2, Lookup - Aero Torque y/2, Lookup - Aero Torque x/2
  Lookup - Aero Torque y/1 -> Mux/2  "Ty BRF"
  Lookup - Aero Torque x/1 -> Mux/1  "Tx BRF"
  Lookup - Aero Torque z/1 -> Mux/3  "Tz BRF"
  Mux/1 -> Product1/2
  Product3/1 -> Product1/1, Scope/1
  Product1/1 -> Aero. Torque [N.m]/1
  Manual Switch/1 -> Scope8/1, Product3/2
  Position (X) [m]/1 -> Get Density/1(<XYZ_ECI>)
  DOY/1 -> Get Density/2(DOY)
  DCM_i2e/1 -> Get Density/3("DCM_i2e ")
  Get Density/2(Density NRLMSISE) -> Manual Switch/2
  Get Density/1(Density Lookup table) -> Manual Switch/1

== system Control_v6_PID/Disturbance Torques/Gravity Gradient Model ==
  note: \tau_{gg}= 3\mu/r^{3} (u_{nadir}\times J* u_{nadir})
  note: (3*mu/Rs^4*) * Rs = (3*mu/Rs^3) * rs
  note: Nadir [body]
  note: position of satellite [ECI]
  note: Nadir unit vector
      | [body]
  note: Anti-nadir [body]
  note: r^4
  "Position (X) [m] " : Inport
  Attitude (DCMi2b) : Inport  Port=2
  3 * mu : Constant  Value=3*3.9860044188e14
  Cross Product : vrlib/Utilities/Cross Product
  Divide : Product  Inputs=*/
  Dot Product = magnitude squared : DotProduct  InputSameDT=on  OutDataTypeStr=Inherit: Inherit via internal rule
  Gain : Gain  Gain=-1
  Gain1 : Gain  Gain=-1
  J : Constant  Value=sat.inertia
  Math Function : Math  Operator=square  SignedPower=on  SaturateOnIntegerOverflow=on
  Product (not cross) : Product  RndMeth=Zero
  Vector Normal : vrlib/Utilities/Normalize Vector  maxzero=0
  product 1 : Product  Multiplication=Matrix(*)  RndMeth=Zero
  product 2 : Product  Multiplication=Matrix(*)  RndMeth=Zero
  Gravity Gradient [N.m] : Outport
  wires:
  Product (not cross)/1 -> Cross Product/1
  Divide/1 -> Product (not cross)/2
  3 * mu/1 -> Divide/1
  Math Function/1 -> Divide/2
  Vector Normal/1 -> Gain/1
  Cross Product/1 -> Gravity Gradient [N.m]/1
  Dot Product = magnitude squared/1 -> Math Function/1
  Gain/1 -> product 2/2
  product 2/1 -> Cross Product/2
  J/1 -> product 2/1
  Attitude (DCMi2b)/1 -> product 1/1
  product 1/1 -> Vector Normal/1, Gain1/1
  Gain1/1 -> Product (not cross)/1
  "Position (X) [m] "/1 -> product 1/2, Dot Product = magnitude squared/2, Dot Product = magnitude squared/1
